simulink model "sbw_treadmill"  (R2022a)
settings: Solver=ode5  StartTime=0.0  StopTime=600  RelTol=1e-3
values from neighbouring files (symbols this model uses):
  Nctrl = length(controls)    [ready_simulink_model.m]
  Ndiff = length(diffStates)    [ready_simulink_model.m]
  Ts = 1/80    (= 0.0125)    [ready_simulink_model.m]
undefined symbols (not defined in the file or in its folder): data, input, Serial_Port, Standard_Devices, UDP_Protocol
libraries: sldrtlib x4, simulink_extras x3, sharedtransform x1
settings Model: Creator=simonas  LastModifiedBy=sudo
settings DebuggingCC: UnconnectedInputMsg=warning  UnconnectedOutputMsg=warning  UnconnectedLineMsg=warning
settings HardwareCC: ProdBitPerLong=64  ProdHWDeviceType=Intel->x86-64 (Linux 64)
settings RTWCC: Description=Simulink Desktop Real-Time  SystemTargetFile=sldrt.tlc  TemplateMakefile=sldrt.tmf  RTWCompilerOptimization=on  DLArmComputeVersion=19.05
settings CodeAppCC: MaxIdLength=95
settings SimulinkDesktopRealTimeCC: TargetLibSuffix=_sldrt.a  TargetPreCompLibLocation=C:\Program Files\MATLAB\R2022a\toolbox\sldrt\lib\win64

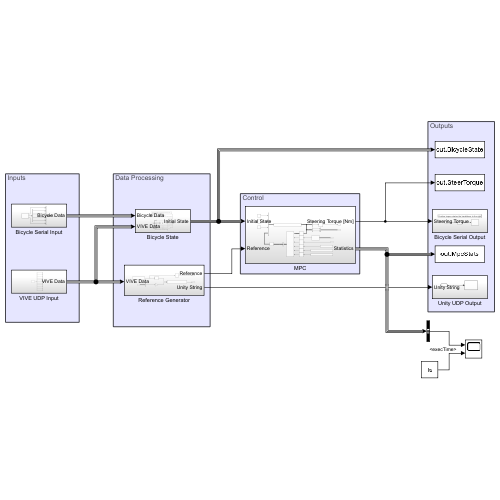
[thumbnail: Simulink's stored preview of the top-level diagram]
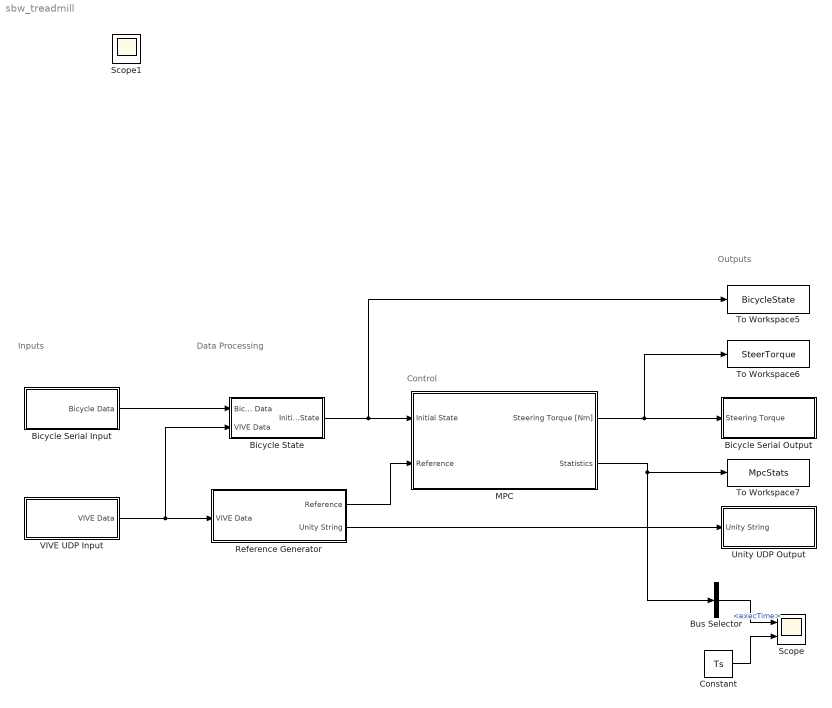
== system sbw_treadmill ==
  note: Control
  note: Data Processing
  note: Inputs
  note: Outputs
  Bicycle Serial Input : Subsystem
  Bicycle Serial Output : Subsystem
  Bicycle State : Subsystem
  Bus Selector : BusSelector  OutputSignals=execTime
  Constant : Constant  Value=Ts  SampleTime=Ts
  MPC : Subsystem
  Reference Generator : Subsystem
  Scope : Scope  NumInputPorts=2
  To Workspace5 : ToWorkspace  VariableName=BicycleState  SaveFormat=Timeseries  SampleTime=-1
  To Workspace6 : ToWorkspace  VariableName=SteerTorque  SaveFormat=Timeseries  SampleTime=-1
  To Workspace7 : ToWorkspace  VariableName=MpcStats  SaveFormat=Timeseries  SampleTime=-1
  Unity UDP Output : Subsystem
  VIVE UDP Input : Subsystem
  Scope1 : Scope
  wires:
  VIVE UDP Input/1(VIVE Data) -> Reference Generator/1(VIVE Data), Bicycle State/2(VIVE Data)
  Reference Generator/1(Reference) -> MPC/2(Reference)
  Bicycle State/1(Initial State) -> To Workspace5/1, MPC/1(Initial State)
  Bicycle Serial Input/1(Bicycle Data) -> Bicycle State/1(Bicycle Data)
  Reference Generator/2(Unity String) -> Unity UDP Output/1(Unity String)
  MPC/2(Statistics) -> Bus Selector/1, To Workspace7/1
  MPC/1(Steering Torque [Nm]) -> To Workspace6/1, Bicycle Serial Output/1(Steering Torque)
  Bus Selector/1 -> Scope/1  "<execTime>"
  Constant/1 -> Scope/2

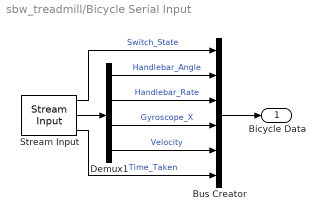
== system sbw_treadmill/Bicycle Serial Input ==
  Bus Creator : BusCreator  Inputs=6
  Demux1 : Demux
  Stream Input : sldrtlib/Stream Input  SampleTime=0.001  MaxMissedTicks=1000000  ShowMissedTicks=off  YieldWhenWaiting=on  DrvName=Standard_Devices/Serial_Port  DrvAddress=4  DrvOptions=[115200 8 0 0 0 0 0 0]  DataTypes={'uint8','4*double','uint32'}  FormatString='%d,%f,%f,%f,%f,%d'  Terminator={'\n'}  ShowReady=off  ShowError=off
      settings: AttributesFormatString=Serial Port [4]  SourceProductBaseCode=WT
  Bicycle Data : Outport
  wires:
  Stream Input/2 -> Demux1/1
  Demux1/2 -> Bus Creator/3  "Handlebar_Rate"
  Stream Input/1 -> Bus Creator/1  "Switch_State"
  Demux1/3 -> Bus Creator/4  "Gyroscope_X"
  Stream Input/3 -> Bus Creator/6  "Time_Taken"
  Demux1/1 -> Bus Creator/2  "Handlebar_Angle"
  Demux1/4 -> Bus Creator/5  "Velocity"
  Bus Creator/1 -> Bicycle Data/1

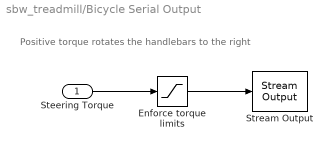
== system sbw_treadmill/Bicycle Serial Output ==
  note: Positive torque rotates the handlebars to the right
  Steering Torque : Inport
  Enforce torque limits : Saturate  UpperLimit=7  LowerLimit=-7
  Stream Output : sldrtlib/Stream Output  SampleTime=0.001  MaxMissedTicks=1000000  ShowMissedTicks=off  YieldWhenWaiting=on  DrvName=Standard_Devices/Serial_Port  DrvAddress=4  DrvOptions=[115200 8 0 0 0 0 0 0]  PortSizes=1  FormatString='%.3f\n'  ShowReady=off  ShowError=off  InitialValue=[]  FinalValue=[]
      settings: AttributesFormatString=Serial Port [4]  SourceProductBaseCode=WT
  wires:
  Steering Torque/1 -> Enforce torque limits/1
  Enforce torque limits/1 -> Stream Output/1

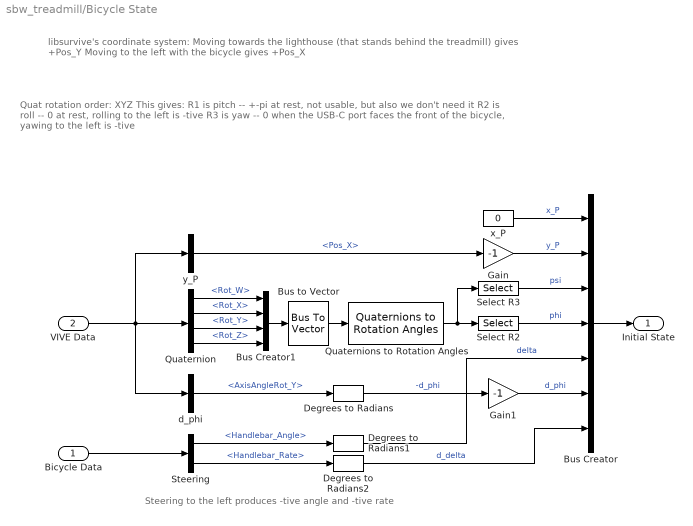
== system sbw_treadmill/Bicycle State ==
  note: Steering to the left produces -tive angle and -tive rate
  note: libsurvive's coordinate system:
      | Moving towards the lighthouse (that stands behind the treadmill) gives +Pos_Y
      | Moving to the left with the bicycle gives +Pos_X
  note: Quat rotation order: XYZ
      | This gives:
      | R1 is pitch -- +-pi at rest, not usable, but also we don't need it
      | R2 is roll -- 0 at rest, rolling to the left is -tive
      | R3 is yaw -- 0 when the USB-C port faces the front of the bicycle, yawing to the left is -tive
  Bicycle Data : Inport
  VIVE Data : Inport  Port=2
  Bus Creator : BusCreator  Inputs=7
  Bus Creator1 : BusCreator  Inputs=4
  Bus to Vector : BusToVector
  Degrees to Radians : simulink_extras/Transformations/Degrees to Radians
  Degrees to Radians1 : simulink_extras/Transformations/Degrees to Radians
  Degrees to Radians2 : simulink_extras/Transformations/Degrees to Radians
  Gain : Gain  Gain=-1
  Gain1 : Gain  Gain=-1
  Quaternion : BusSelector  OutputSignals=Rot_W,Rot_X,Rot_Y,Rot_Z
  Quaternions to Rotation Angles : sharedtransform/Quaternions to Rotation Angles  rotationOrder=XYZ  aMode=aMode
      settings: SourceProductBaseCode=AE,PW,DR,MT,VE
  Select R2 : Selector  InputPortWidth=3  IndexOptions=Index vector (dialog)  Indices=2  OutputSizes=1
  Select R3 : Selector  InputPortWidth=3  IndexOptions=Index vector (dialog)  Indices=3  OutputSizes=1
  Steering : BusSelector  OutputSignals=Handlebar_Angle,Handlebar_Rate
  d_phi : BusSelector  OutputSignals=AxisAngleRot_Y
  x_P : Constant  Value=0
  y_P : BusSelector  OutputSignals=Pos_X
  Initial State : Outport
  wires:
  x_P/1 -> Bus Creator/1  "x_P"
  VIVE Data/1 -> d_phi/1, y_P/1, Quaternion/1
  Quaternion/2 -> Bus Creator1/2  "<Rot_X>"
  Quaternion/3 -> Bus Creator1/3  "<Rot_Y>"
  Quaternion/4 -> Bus Creator1/4  "<Rot_Z>"
  Select R3/1 -> Bus Creator/3  "psi"
  Select R2/1 -> Bus Creator/4  "phi"
  d_phi/1 -> Degrees to Radians/1  "<AxisAngleRot_Y>"
  y_P/1 -> Gain/1  "<Pos_X>"
  Bicycle Data/1 -> Steering/1
  Steering/1 -> Degrees to Radians1/1  "<Handlebar_Angle>"
  Steering/2 -> Degrees to Radians2/1  "<Handlebar_Rate>"
  Bus Creator/1 -> Initial State/1
  Quaternion/1 -> Bus Creator1/1  "<Rot_W>"
  Bus Creator1/1 -> Bus to Vector/1
  Bus to Vector/1 -> Quaternions to Rotation Angles/1
  Quaternions to Rotation Angles/1 -> Select R2/1, Select R3/1
  Degrees to Radians/1 -> Gain1/1  "-d_phi"
  Degrees to Radians1/1 -> Bus Creator/5  "delta"
  Degrees to Radians2/1 -> Bus Creator/7  "d_delta"
  Gain/1 -> Bus Creator/2  "y_P"
  Gain1/1 -> Bus Creator/6  "d_phi"

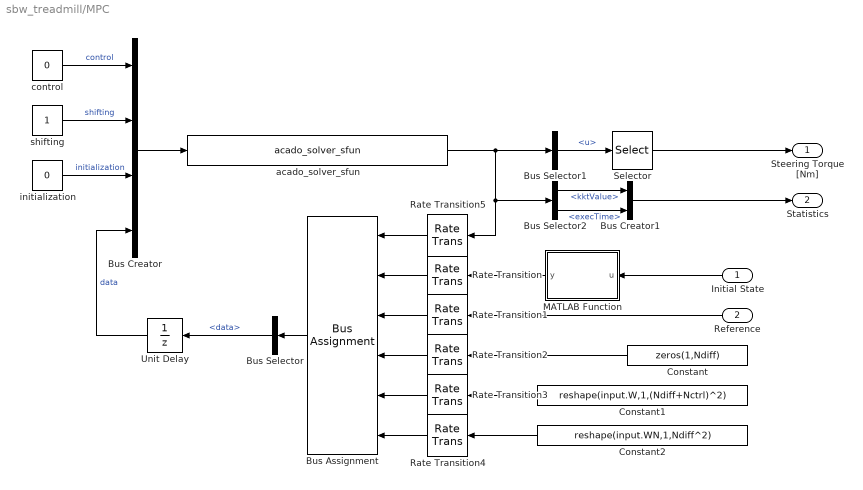
== system sbw_treadmill/MPC ==
  Initial State : Inport
  Reference : Inport  Port=2
  Bus Assignment : BusAssignment  AssignedSignals=data.x0,data.y,data.yN,data.W,data.WN
  Bus Creator : BusCreator  Inputs=4
  Bus Creator1 : BusCreator  Inputs=2
  Bus Selector : BusSelector  OutputSignals=data
  Bus Selector1 : BusSelector  OutputSignals=data.u
  Bus Selector2 : BusSelector  OutputSignals=kktValue,execTime
  Constant : Constant  Value=zeros(1,Ndiff)
  Constant1 : Constant  Value=reshape(input.W,1,(Ndiff+Nctrl)^2)
  Constant2 : Constant  Value=reshape(input.WN,1,Ndiff^2)
  MATLAB Function : MATLAB Function  TreatAsAtomicUnit=on  SystemSampleTime=Ts
  Rate Transition{,1..5} (6 alike) : RateTransition  OutPortSampleTime=Ts
  Selector : Selector  InputPortWidth=Nhorizon  IndexOptions=Index vector (dialog)  Indices=[1]  OutputSizes=1
  Unit Delay : UnitDelay  SampleTime=Ts  HasFrameUpgradeWarning=on
  acado_solver_sfun : S-Function  FunctionName=acado_solver_sfun  SFunctionDeploymentMode=off  EnableBusSupport=off  mask(Legacy Function){SFunctionSpec=acado_step(ACADOinput u1[1], ACADOoutput y1[1]), ShowSpec=on}
      mask prompts: ShowSpec "Display function specification"
      mask help:
      | This block allows you to call the legacy functions specified by the following Legacy Code Tool definition:
      | def.SFunctionName = 'acado_solver_sfun';
      | def.OutputFcnSpec = 'acado_step(ACADOinput u1[1], ACADOoutput y1[1])';
      | def.StartFcnSpec = 'acado_initialize( void )';
      | def.TerminateFcnSpec = 'acado_cleanup( void )';
      | def.HeaderFiles = {'acado_common.h', 'acado_solver_sfunction.h'};
      | def.SourceFiles = {'acado_solver.c', 'acado_integrator.c', 'acado_auxiliary_functions.c', 'acado_solver_sfunction.c', 'acado_qpoases3_interface.c', 'qpoases3\src\Bounds.c', 'qpoases3\src\Constraints.c', 'qpoases3\src\Indexlist.c', 'qpoases3\src\Matrices.c', 'qpoases3\src\MessageHandling.c', 'qpoases3\src\Options.c', 'qpoases3\src\Flipper.c', 'qpoases3\src\QProblem.c', 'qpoases3\src\QProblemB.c', 'qpoases3\src\Utils.c'};
      mask Help: <p>This block was generated automatically by the Legacy Code Tool. For detailed help on this tool, call<a href="matlab:legacy_code('help')"> legacy_code('help')</a>.</p>
      mask Callback ShowSpec:
      | if strcmp(get_param(gcbh, 'ShowSpec'), 'on')
      |   set_param(gcbh, 'MaskDisplay', sprintf('fprintf(''%s'');', get_param(gcbh, 'SFunctionSpec')));
      | else
      |   set_param(gcbh, 'MaskDisplay', sprintf('fprintf(''%s'');', get_param(gcbh, 'FunctionName')));
      | end
      mask Display: fprintf('acado_step(ACADOinput u1[1], ACADOoutput y1[1])');
  control : Constant  Value=0  OutDataTypeStr=int32
  initialization : Constant  Value=0  OutDataTypeStr=int32
  shifting : Constant  OutDataTypeStr=int32
  Steering Torque [Nm] : Outport
  Statistics : Outport  Port=2
  wires:
  Bus Creator/1 -> acado_solver_sfun/1
  initialization/1 -> Bus Creator/3  "initialization"
  Bus Assignment/1 -> Bus Selector/1
  acado_solver_sfun/1 -> Bus Selector1/1, Rate Transition5/1, Bus Selector2/1
  shifting/1 -> Bus Creator/2  "shifting"
  Bus Selector2/1 -> Bus Creator1/1  "<kktValue>"
  Initial State/1 -> MATLAB Function/1(u)
  Bus Creator1/1 -> Statistics/1
  Unit Delay/1 -> Bus Creator/4  "data"
  control/1 -> Bus Creator/1  "control"
  Bus Selector1/1 -> Selector/1  "<u>"
  Bus Selector2/2 -> Bus Creator1/2  "<execTime>"
  Bus Selector/1 -> Unit Delay/1  "<data>"
  MATLAB Function/1(y) -> Rate Transition/1
  Rate Transition/1 -> Bus Assignment/2
  Rate Transition1/1 -> Bus Assignment/3
  Reference/1 -> Rate Transition1/1
  Constant/1 -> Rate Transition2/1
  Rate Transition2/1 -> Bus Assignment/4
  Constant1/1 -> Rate Transition3/1
  Rate Transition3/1 -> Bus Assignment/5
  Constant2/1 -> Rate Transition4/1
  Rate Transition4/1 -> Bus Assignment/6
  Rate Transition5/1 -> Bus Assignment/1
  Selector/1 -> Steering Torque [Nm]/1

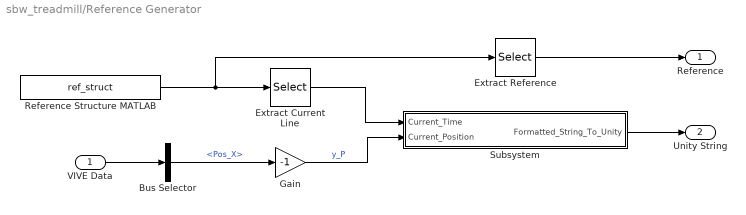
== system sbw_treadmill/Reference Generator ==
  VIVE Data : Inport
  Bus Selector : BusSelector  OutputSignals=Pos_X
  Extract Current Line : Selector  InputPortWidth=1281  IndexOptions=Index vector (dialog)  Indices=1  OutputSizes=1
  Extract Reference : Selector  InputPortWidth=1281  IndexOptions=Index vector (dialog)  Indices=2:1281  OutputSizes=1
  Gain : Gain  Gain=-1
  Reference Structure MATLAB : FromWorkspace  VariableName=ref_struct  SampleTime=Ts  Interpolate=off  ZeroCross=off  OutputAfterFinalValue=Cyclic repetition
  Subsystem : Subsystem
  Reference : Outport
  Unity String : Outport  Port=2  OutDataTypeStr=string
  wires:
  Subsystem/1(Formatted_String_To_Unity) -> Unity String/1
  Reference Structure MATLAB/1 -> Extract Reference/1, Extract Current Line/1
  Extract Current Line/1 -> Subsystem/1(Current_Time)
  VIVE Data/1 -> Bus Selector/1
  Bus Selector/1 -> Gain/1  "<Pos_X>"
  Extract Reference/1 -> Reference/1
  Gain/1 -> Subsystem/2(Current_Position)  "y_P"

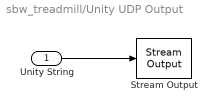
== system sbw_treadmill/Unity UDP Output ==
  Unity String : Inport
  Stream Output : sldrtlib/Stream Output  SampleTime=0.001  MaxMissedTicks=1000000  ShowMissedTicks=off  YieldWhenWaiting=on  DrvName=Standard_Devices/UDP_Protocol  DrvAddress=8005  DrvOptions=[0 8006 49 50 55 46 48 46 48 46 49 0 0 0 0 0 0 0 0 0 0 0 0 0 0 0 0 0 0 0 0 0 0 0 0 0 0 0 0 0 0 0 0 0 0 0 0 0 0 0 0 0 0 0 0 0 0 0 0 0 0 0 0 0 0 0 0 0 0 0 0 0 0 0 0 0 0 0 0 0 0 0 0 0 0 0 0 0 0 0 0 0 0 0 0 0 0 0 0 0 0 0 0 0 0 0 0 0 0 0 0 0 0 0 0 0 0 0 0 0 0 0 0 0 0 0 0 0 0 0 0 0 0 0 0 0 0 0 0 0 0 0 0 0 0 0 0 0 0 0 0 0 0 0 0 0 0 0 0 0 0 0 0 0 0 0 0 0 0 0 0 0 0 0 0 0 0 0 0 0 0 0 0 0 0 0 0 0 0 0 0 0 0 0 0 0 0 0 0 0 0 0 0 0 0 0 0 0 0 0 0 0 0 0 0 0 0 0 0 0 0 0 0 0 0 0 0 0 0 0 0 0 0 0 0 0 0 0 0 0 0 0 0 0 0 0 0 0 0 0 0 0 0 0 0 0]  PortSizes=1  FormatString='%s'  ShowReady=off  ShowError=off  InitialValue=[]  FinalValue=[]
      settings: AttributesFormatString=UDP Protocol [8005]  SourceProductBaseCode=WT
  wires:
  Unity String/1 -> Stream Output/1

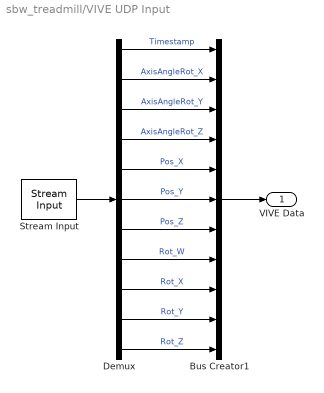
== system sbw_treadmill/VIVE UDP Input ==
  Bus Creator1 : BusCreator  Inputs=11
  Demux : Demux  Outputs=11
  Stream Input : sldrtlib/Stream Input  SampleTime=0.004  MaxMissedTicks=1000000  ShowMissedTicks=off  YieldWhenWaiting=on  DrvName=Standard_Devices/UDP_Protocol  DrvAddress=4950  DrvOptions=[0 16385 0 0 0 0 0 0 0 0 0 0 0 0 0 0 0 0 0 0 0 0 0 0 0 0 0 0 0 0 0 0 0 0 0 0 0 0 0 0 0 0 0 0 0 0 0 0 0 0 0 0 0 0 0 0 0 0 0 0 0 0 0 0 0 0 0 0 0 0 0 0 0 0 0 0 0 0 0 0 0 0 0 0 0 0 0 0 0 0 0 0 0 0 0 0 0 0 0 0 0 0 0 0 0 0 0 0 0 0 0 0 0 0 0 0 0 0 0 0 0 0 0 0 0 0 0 0 0 0 0 0 0 0 0 0 0 0 0 0 0 0 0 0 0 0 0 0 0 0 0 0 0 0 0 0 0 0 0 0 0 0 0 0 0 0 0 0 0 0 0 0 0 0 0 0 0 0 0 0 0 0 0 0 0 0 0 0 0 0 0 0 0 0 0 0 0 0 0 0 0 0 0 0 0 0 0 0 0 0 0 0 0 0 0 0 0 0 0 0 0 0 0 0 0 0 0 0 0 0 0 0 0 0 0 0 0 0 0 0 0 0 0 0 0 0 0 0 0 0 0 0 0 0 0 0]  DataTypes={'11*double'}  FormatString='%f,%f,%f,%f,%f,%f,%f,%f,%f,%f,%f'  Terminator='\n'  ShowReady=off  ShowError=off
      settings: AttributesFormatString=UDP Protocol [4950]  SourceProductBaseCode=WT
  VIVE Data : Outport
  wires:
  Demux/7 -> Bus Creator1/7  "Pos_Z"
  Demux/8 -> Bus Creator1/8  "Rot_W"
  Stream Input/1 -> Demux/1
  Demux/10 -> Bus Creator1/10  "Rot_Y"
  Bus Creator1/1 -> VIVE Data/1
  Demux/9 -> Bus Creator1/9  "Rot_X"
  Demux/1 -> Bus Creator1/1  "Timestamp"
  Demux/4 -> Bus Creator1/4  "AxisAngleRot_Z"
  Demux/3 -> Bus Creator1/3  "AxisAngleRot_Y"
  Demux/5 -> Bus Creator1/5  "Pos_X"
  Demux/2 -> Bus Creator1/2  "AxisAngleRot_X"
  Demux/11 -> Bus Creator1/11  "Rot_Z"
  Demux/6 -> Bus Creator1/6  "Pos_Y"

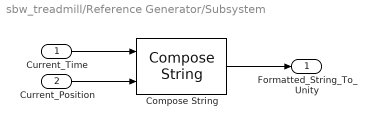
== system sbw_treadmill/Reference Generator/Subsystem ==
  Current_Time : Inport
  Current_Position : Inport  Port=2
  Compose String : ComposeString  Format="\"%.0f,%.3f\\n\""
  Formatted_String_To_Unity : Outport
  wires:
  Current_Position/1 -> Compose String/2
  Compose String/1 -> Formatted_String_To_Unity/1
  Current_Time/1 -> Compose String/1

== matlab function sbw_treadmill/MPC/MATLAB Function ==
  data: u input; y output
function y = fcn(u)
    
y = u';
